simulink model "airplaneFlightController_mdl"  (R2022b)
settings: Solver=ode4  StartTime=0.0  StopTime=10  FixedStep=.001  RelTol=1e-3
undefined symbols (not defined in the file): F, G, G_f, G_updated, M, P_0
settings Model: Creator=mo780715  LastModifiedBy=mo780715

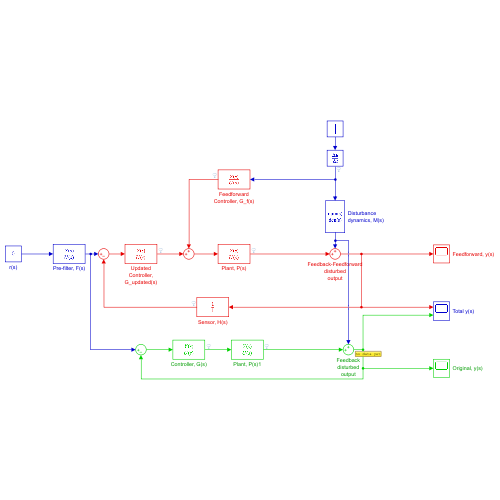
[thumbnail: Simulink's stored preview of the top-level diagram]
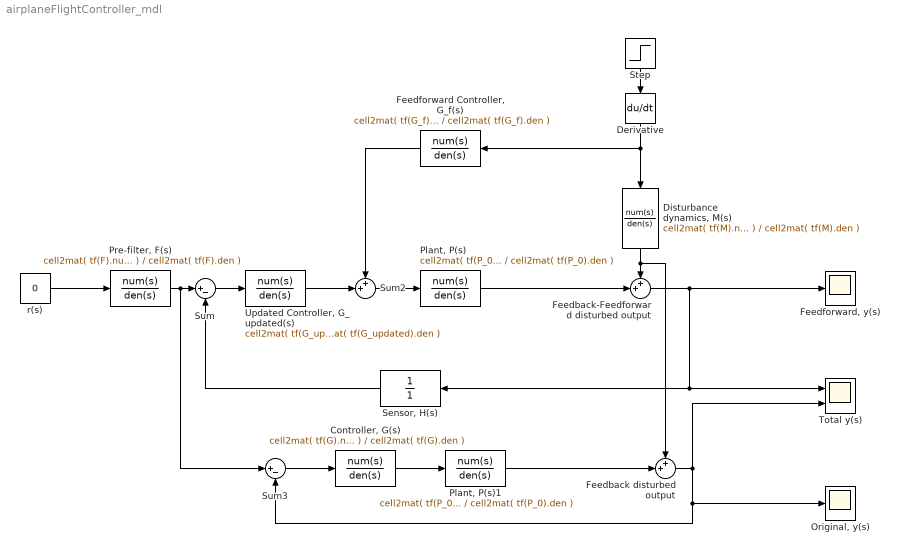
== system airplaneFlightController_mdl ==
  "Controller, G(s)" : TransferFcn  Numerator=cell2mat( tf(G).num )  Denominator=cell2mat( tf(G).den )
  Derivative : Derivative
  "Disturbance dynamics, M(s)" : TransferFcn  Numerator=cell2mat( tf(M).num )  Denominator=cell2mat( tf(M).den )
  Feedback disturbed output : Sum  Inputs=++|
  Feedback-Feedforward disturbed output : Sum  Inputs=++|
  "Feedforward Controller, G_f(s)" : TransferFcn  Numerator=cell2mat( tf(G_f).num )  Denominator=cell2mat( tf(G_f).den )
  "Feedforward, y(s)" : Scope
  "Original, y(s)" : Scope
  "Plant, P(s)" : TransferFcn  Numerator=cell2mat( tf(P_0).num )  Denominator=cell2mat( tf(P_0).den )
  "Plant, P(s)1" : TransferFcn  Numerator=cell2mat( tf(P_0).num )  Denominator=cell2mat( tf(P_0).den )
  "Pre-filter, F(s)" : TransferFcn  Numerator=cell2mat( tf(F).num )  Denominator=cell2mat( tf(F).den )
  "Sensor, H(s)" : TransferFcn  Numerator=1  Denominator=1
  Step : Step  SampleTime=0
  Sum : Sum  Inputs=|+-
  Sum2 : Sum  Inputs=++|
  Sum3 : Sum  Inputs=|+-
  Total y(s) : Scope  NumInputPorts=2
  "Updated Controller, G_updated(s)" : TransferFcn  Numerator=cell2mat( tf(G_updated).num )  Denominator=cell2mat( tf(G_updated).den )
  r(s) : Constant  Value=0
  wires:
  Feedback-Feedforward disturbed output/1 -> "Sensor, H(s)"/1, Total y(s)/1, "Feedforward, y(s)"/1
  "Plant, P(s)"/1 -> Feedback-Feedforward disturbed output/2
  r(s)/1 -> "Pre-filter, F(s)"/1
  "Pre-filter, F(s)"/1 -> Sum3/1, Sum/1
  Sum/1 -> "Updated Controller, G_updated(s)"/1
  "Disturbance dynamics, M(s)"/1 -> Feedback disturbed output/1, Feedback-Feedforward disturbed output/1
  Step/1 -> Derivative/1
  "Updated Controller, G_updated(s)"/1 -> Sum2/2
  Sum2/1 -> "Plant, P(s)"/1
  "Feedforward Controller, G_f(s)"/1 -> Sum2/1
  "Sensor, H(s)"/1 -> Sum/2
  Derivative/1 -> "Disturbance dynamics, M(s)"/1, "Feedforward Controller, G_f(s)"/1
  "Controller, G(s)"/1 -> "Plant, P(s)1"/1
  Sum3/1 -> "Controller, G(s)"/1
  "Plant, P(s)1"/1 -> Feedback disturbed output/2
  Feedback disturbed output/1 -> Sum3/2, "Original, y(s)"/1, Total y(s)/2
